simulink model "modello"  (R2023b)
settings: Solver=VariableStepAuto  StartTime=0.0  StopTime=150  RelTol=1e-3
undefined symbols (not defined in the file or in its folder): properties
libraries: fl_lib x60, nesl_utility x27, simulink x1
settings Model: Creator=brent  LastModifiedBy=brent

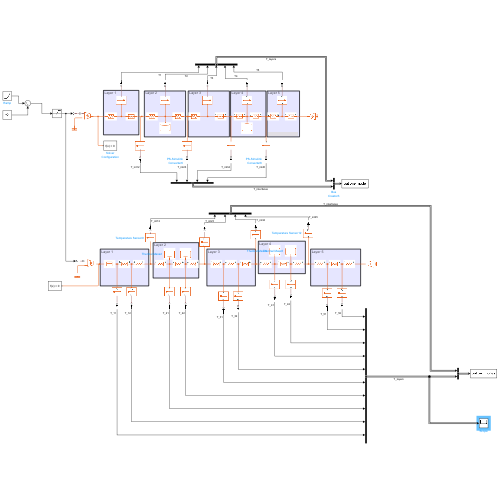
[thumbnail: Simulink's stored preview of the top-level diagram]
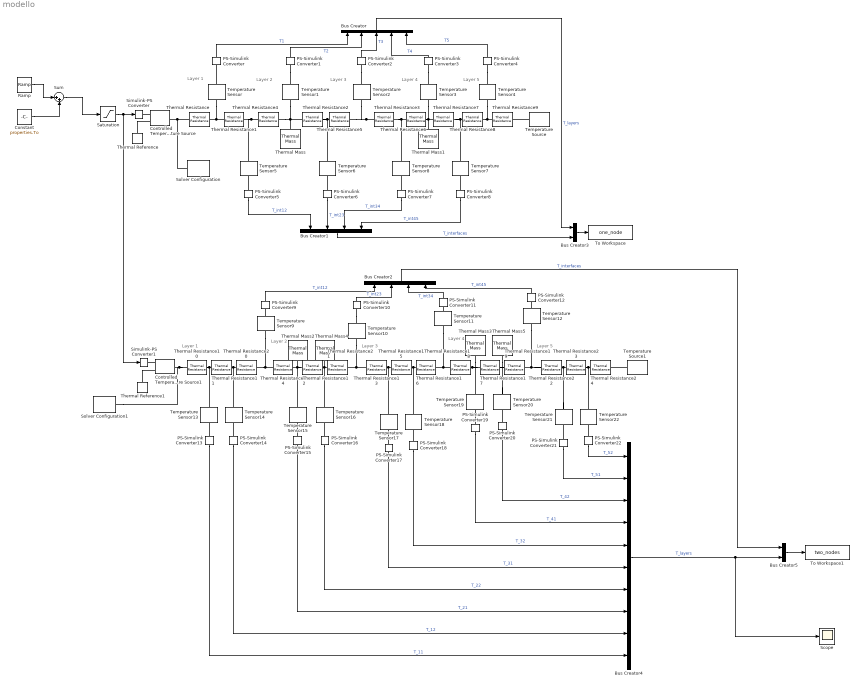
== system modello ==
  note: Layer 1
  note: Layer 2
  note: Layer 1
  note: Layer 3
  note: Layer 4
  note: Layer 5
  note: Layer 2
  note: Layer 3
  note: Layer 4
  note: Layer 5
  Bus Creator : BusCreator  Inputs=5
  Bus Creator1 : BusCreator  Inputs=4
  Bus Creator2 : BusCreator  Inputs=4
  Bus Creator3 : BusCreator  Inputs=2
  Bus Creator4 : BusCreator  Inputs=10
  Bus Creator5 : BusCreator  Inputs=2
  Constant : Constant  Value=properties.To
  Controlled Temperature Source : fl_lib/Thermal/Thermal Sources/Controlled Temperature Source
  Controlled Temperature Source1 : fl_lib/Thermal/Thermal Sources/Controlled Temperature Source
  PS-Simulink Converter{,1..22} (23 alike) : nesl_utility/PS-Simulink Converter  PhysicalDomain=network_engine_domain  SubClassName=ps_output  LeftPortType=input  RightPortType=output  PseudoPeriodic=off  Frequencies=[]  VectorFormat=inherit  Unit=inherit  AffineConversion=off
  Ramp : simulink/Sources/Ramp  slope=980+ 273.15  start=0  InitialOutput=0
  Saturation : Saturate  UpperLimit=1273.15  LowerLimit=273
  Scope : Scope
  Simulink-PS Converter : nesl_utility/Simulink-PS Converter  PhysicalDomain=network_engine_domain  SubClassName=ps_input  LeftPortType=input  RightPortType=output  PseudoPeriodic=off  Frequencies=[]  NoiseDistribution=none  NoiseParameters=[]  Unit=1  AffineConversion=off  FilteringAndDerivatives=provide  SimscapeFilterOrder=1  InputFilterTimeConstant=0.001  UdotUserProvided=0
  Simulink-PS Converter1 : nesl_utility/Simulink-PS Converter  PhysicalDomain=network_engine_domain  SubClassName=ps_input  LeftPortType=input  RightPortType=output  PseudoPeriodic=off  Frequencies=[]  NoiseDistribution=none  NoiseParameters=[]  Unit=1  AffineConversion=off  FilteringAndDerivatives=provide  SimscapeFilterOrder=1  InputFilterTimeConstant=0.001  UdotUserProvided=0
  Solver Configuration : nesl_utility/Solver Configuration  PhysicalDomain=network_engine_domain  SubClassName=solver  LeftPortType=input  RightPortType=generic  Tones=[]  Harmonics=[]  SimulateNoise=off  Profile=off  UseLocalSampling=off  EnableSwitchedLinearOptims=on  FrequencyDomain=off  UseCCode=off  RelTol=0.001  AbsTol=0.001  MinStep=1e-09  ToWorkspace=off  RevertToSquareIcSolve=off  NumHomotopyIterations=100  PhasorMode=off  PhasorModeNumHarmonics=1  ConsistencySolver=NEWTON_XTOL_AFTER_FTOL  IndexReductionMethod=DerivativeReplacement  DoDC=on  ResidualTolerance=1e-09  ConsistencyTolSource=GLOBAL  ConsistencyAbsTol=0.001  ConsistencyRelTol=0.001  ConsistencyTolFactor=ode_tol  UseLocalSolver=off  LocalSolverChoice=NE_BACKWARD_EULER_ADVANCER  ResolveIndetEquations=on  FunctionEvalNumThread=1  LocalSolverSampleTime=0.001  DoFixedCost=off  MaxNonlinIter=3  MaxModeIter=2  ComputeImpulses=off  ImpulseIterations=2  LinearAlgebra=auto  LinearAlgebraNumThread=0  EquationFormulation=NE_TIME_EF  DelaysMemoryBudget=1024  AutomaticFiltering=off  FilteringTimeConstant=0.001  PartitionStorageMethod=AS_NEEDED  PartitionMemoryBudget=1024  PartitionMethod=ROBUST  MultibodyUseLocalSolver=off  MultibodyLocalSolverChoice=ODE1  MultibodyLocalSolverSampleTime=0.001
  Solver Configuration1 : nesl_utility/Solver Configuration  PhysicalDomain=network_engine_domain  SubClassName=solver  LeftPortType=input  RightPortType=generic  Tones=[]  Harmonics=[]  SimulateNoise=off  Profile=off  UseLocalSampling=off  EnableSwitchedLinearOptims=on  FrequencyDomain=off  UseCCode=off  RelTol=0.001  AbsTol=0.001  MinStep=1e-09  ToWorkspace=off  RevertToSquareIcSolve=off  NumHomotopyIterations=100  PhasorMode=off  PhasorModeNumHarmonics=1  ConsistencySolver=NEWTON_XTOL_AFTER_FTOL  IndexReductionMethod=DerivativeReplacement  DoDC=on  ResidualTolerance=1e-09  ConsistencyTolSource=GLOBAL  ConsistencyAbsTol=0.001  ConsistencyRelTol=0.001  ConsistencyTolFactor=ode_tol  UseLocalSolver=off  LocalSolverChoice=NE_BACKWARD_EULER_ADVANCER  ResolveIndetEquations=on  FunctionEvalNumThread=1  LocalSolverSampleTime=0.001  DoFixedCost=off  MaxNonlinIter=3  MaxModeIter=2  ComputeImpulses=off  ImpulseIterations=2  LinearAlgebra=auto  LinearAlgebraNumThread=0  EquationFormulation=NE_TIME_EF  DelaysMemoryBudget=1024  AutomaticFiltering=off  FilteringTimeConstant=0.001  PartitionStorageMethod=AS_NEEDED  PartitionMemoryBudget=1024  PartitionMethod=ROBUST  MultibodyUseLocalSolver=off  MultibodyLocalSolverChoice=ODE1  MultibodyLocalSolverSampleTime=0.001
  Sum : Sum  Inputs=|++
  Temperature Sensor{,1..22} (23 alike) : fl_lib/Thermal/Thermal Sensors/Temperature Sensor  temperature_measure=foundation.enum.MeasurementReference.absolute
      settings: InternalSimscapePortConfiguration="{\"Bottom\":[],\"Left\":[{\"id\":\"A\",\"label\":\"A\",\"type\":\"foundation.thermal.thermal\"}],\"Right\":[{\"id\":\"T\",\"label\":\"T\",\"type\":\"output\"}],\"Top\":[]}"
  Temperature Source : fl_lib/Thermal/Thermal Sources/Temperature Source  temperature=293.15 K
  Temperature Source1 : fl_lib/Thermal/Thermal Sources/Temperature Source  temperature=293.15 K
  Thermal Mass : fl_lib/Thermal/Thermal Elements/Thermal Mass  mass_type=foundation.enum.constant_variable.constant  mass=1 kg  sp_heat=properties.C2 J/(K*kg)  mass_min=1e-6 kg  num_ports=foundation.enum.numPorts2.one  m_specify=off  m_priority=High  m=1 kg  m_nominal_specify=off  m_nominal_unit=kg  m_nominal_value=1  T_specify=off  T_priority=High  T=300 K  T_nominal_specify=off  T_nominal_unit=K  T_nominal_value=1  Q_specify=off  Q_priority=None  Q=0 W  Q_nominal_specify=off  Q_nominal_unit=W  Q_nominal_value=1
  Thermal Mass1 : fl_lib/Thermal/Thermal Elements/Thermal Mass  mass_type=foundation.enum.constant_variable.constant  mass=1 kg  sp_heat=properties.C4 J/(K*kg)  mass_min=1e-6 kg  num_ports=foundation.enum.numPorts2.one  m_specify=off  m_priority=High  m=1 kg  m_nominal_specify=off  m_nominal_unit=kg  m_nominal_value=1  T_specify=off  T_priority=High  T=300 K  T_nominal_specify=off  T_nominal_unit=K  T_nominal_value=1  Q_specify=off  Q_priority=None  Q=0 W  Q_nominal_specify=off  Q_nominal_unit=W  Q_nominal_value=1
  Thermal Mass2 : fl_lib/Thermal/Thermal Elements/Thermal Mass  mass_type=foundation.enum.constant_variable.constant  mass=1 kg  sp_heat=properties.C2/2 J/(K*kg)  mass_min=1e-6 kg  num_ports=foundation.enum.numPorts2.one  m_specify=off  m_priority=High  m=1 kg  m_nominal_specify=off  m_nominal_unit=kg  m_nominal_value=1  T_specify=off  T_priority=High  T=300 K  T_nominal_specify=off  T_nominal_unit=K  T_nominal_value=1  Q_specify=off  Q_priority=None  Q=0 W  Q_nominal_specify=off  Q_nominal_unit=W  Q_nominal_value=1
  Thermal Mass3 : fl_lib/Thermal/Thermal Elements/Thermal Mass  mass_type=foundation.enum.constant_variable.constant  mass=1 kg  sp_heat=properties.C4/2 J/(K*kg)  mass_min=1e-6 kg  num_ports=foundation.enum.numPorts2.one  m_specify=off  m_priority=High  m=1 kg  m_nominal_specify=off  m_nominal_unit=kg  m_nominal_value=1  T_specify=off  T_priority=High  T=300 K  T_nominal_specify=off  T_nominal_unit=K  T_nominal_value=1  Q_specify=off  Q_priority=None  Q=0 W  Q_nominal_specify=off  Q_nominal_unit=W  Q_nominal_value=1
  Thermal Mass4 : fl_lib/Thermal/Thermal Elements/Thermal Mass  mass_type=foundation.enum.constant_variable.constant  mass=1 kg  sp_heat=properties.C2/2 J/(K*kg)  mass_min=1e-6 kg  num_ports=foundation.enum.numPorts2.one  m_specify=off  m_priority=High  m=1 kg  m_nominal_specify=off  m_nominal_unit=kg  m_nominal_value=1  T_specify=off  T_priority=High  T=300 K  T_nominal_specify=off  T_nominal_unit=K  T_nominal_value=1  Q_specify=off  Q_priority=None  Q=0 W  Q_nominal_specify=off  Q_nominal_unit=W  Q_nominal_value=1
  Thermal Mass5 : fl_lib/Thermal/Thermal Elements/Thermal Mass  mass_type=foundation.enum.constant_variable.constant  mass=1 kg  sp_heat=properties.C4/2 J/(K*kg)  mass_min=1e-6 kg  num_ports=foundation.enum.numPorts2.one  m_specify=off  m_priority=High  m=1 kg  m_nominal_specify=off  m_nominal_unit=kg  m_nominal_value=1  T_specify=off  T_priority=High  T=300 K  T_nominal_specify=off  T_nominal_unit=K  T_nominal_value=1  Q_specify=off  Q_priority=None  Q=0 W  Q_nominal_specify=off  Q_nominal_unit=W  Q_nominal_value=1
  Thermal Reference : fl_lib/Thermal/Thermal Elements/Thermal Reference
  Thermal Reference1 : fl_lib/Thermal/Thermal Elements/Thermal Reference
  Thermal Resistance : fl_lib/Thermal/Thermal Elements/Thermal Resistance  resistance=properties.R1/2 K/W  T_specify=off  T_priority=None  T=0 K  T_nominal_specify=off  T_nominal_unit=K  T_nominal_value=1  Q_specify=off  Q_priority=None  Q=0 W  Q_nominal_specify=off  Q_nominal_unit=W  Q_nominal_value=1
  Thermal Resistance1 : fl_lib/Thermal/Thermal Elements/Thermal Resistance  resistance=properties.R1/2 K/W  T_specify=off  T_priority=None  T=0 K  T_nominal_specify=off  T_nominal_unit=K  T_nominal_value=1  Q_specify=off  Q_priority=None  Q=0 W  Q_nominal_specify=off  Q_nominal_unit=W  Q_nominal_value=1
  Thermal Resistance10 : fl_lib/Thermal/Thermal Elements/Thermal Resistance  resistance=properties.R1/3 K/W  T_specify=off  T_priority=None  T=0 K  T_nominal_specify=off  T_nominal_unit=K  T_nominal_value=1  Q_specify=off  Q_priority=None  Q=0 W  Q_nominal_specify=off  Q_nominal_unit=W  Q_nominal_value=1
  Thermal Resistance11 : fl_lib/Thermal/Thermal Elements/Thermal Resistance  resistance=properties.R1/3 K/W  T_specify=off  T_priority=None  T=0 K  T_nominal_specify=off  T_nominal_unit=K  T_nominal_value=1  Q_specify=off  Q_priority=None  Q=0 W  Q_nominal_specify=off  Q_nominal_unit=W  Q_nominal_value=1
  Thermal Resistance12 : fl_lib/Thermal/Thermal Elements/Thermal Resistance  resistance=properties.R2/3 K/W  T_specify=off  T_priority=None  T=0 K  T_nominal_specify=off  T_nominal_unit=K  T_nominal_value=1  Q_specify=off  Q_priority=None  Q=0 W  Q_nominal_specify=off  Q_nominal_unit=W  Q_nominal_value=1
  Thermal Resistance13 : fl_lib/Thermal/Thermal Elements/Thermal Resistance  resistance=properties.R3/3 K/W  T_specify=off  T_priority=None  T=0 K  T_nominal_specify=off  T_nominal_unit=K  T_nominal_value=1  Q_specify=off  Q_priority=None  Q=0 W  Q_nominal_specify=off  Q_nominal_unit=W  Q_nominal_value=1
  Thermal Resistance14 : fl_lib/Thermal/Thermal Elements/Thermal Resistance  resistance=properties.R2/3 K/W  T_specify=off  T_priority=None  T=0 K  T_nominal_specify=off  T_nominal_unit=K  T_nominal_value=1  Q_specify=off  Q_priority=None  Q=0 W  Q_nominal_specify=off  Q_nominal_unit=W  Q_nominal_value=1
  Thermal Resistance15 : fl_lib/Thermal/Thermal Elements/Thermal Resistance  resistance=properties.R3/3 K/W  T_specify=off  T_priority=None  T=0 K  T_nominal_specify=off  T_nominal_unit=K  T_nominal_value=1  Q_specify=off  Q_priority=None  Q=0 W  Q_nominal_specify=off  Q_nominal_unit=W  Q_nominal_value=1
  Thermal Resistance16 : fl_lib/Thermal/Thermal Elements/Thermal Resistance  resistance=properties.R3/3 K/W  T_specify=off  T_priority=None  T=0 K  T_nominal_specify=off  T_nominal_unit=K  T_nominal_value=1  Q_specify=off  Q_priority=None  Q=0 W  Q_nominal_specify=off  Q_nominal_unit=W  Q_nominal_value=1
  Thermal Resistance17 : fl_lib/Thermal/Thermal Elements/Thermal Resistance  resistance=properties.R4/3 K/W  T_specify=off  T_priority=None  T=0 K  T_nominal_specify=off  T_nominal_unit=K  T_nominal_value=1  Q_specify=off  Q_priority=None  Q=0 W  Q_nominal_specify=off  Q_nominal_unit=W  Q_nominal_value=1
  Thermal Resistance18 : fl_lib/Thermal/Thermal Elements/Thermal Resistance  resistance=properties.R4/3 K/W  T_specify=off  T_priority=None  T=0 K  T_nominal_specify=off  T_nominal_unit=K  T_nominal_value=1  Q_specify=off  Q_priority=None  Q=0 W  Q_nominal_specify=off  Q_nominal_unit=W  Q_nominal_value=1
  Thermal Resistance19 : fl_lib/Thermal/Thermal Elements/Thermal Resistance  resistance=properties.R4/3 K/W  T_specify=off  T_priority=None  T=0 K  T_nominal_specify=off  T_nominal_unit=K  T_nominal_value=1  Q_specify=off  Q_priority=None  Q=0 W  Q_nominal_specify=off  Q_nominal_unit=W  Q_nominal_value=1
  Thermal Resistance2 : fl_lib/Thermal/Thermal Elements/Thermal Resistance  resistance=properties.R2/2 K/W  T_specify=off  T_priority=None  T=0 K  T_nominal_specify=off  T_nominal_unit=K  T_nominal_value=1  Q_specify=off  Q_priority=None  Q=0 W  Q_nominal_specify=off  Q_nominal_unit=W  Q_nominal_value=1
  Thermal Resistance20 : fl_lib/Thermal/Thermal Elements/Thermal Resistance  resistance=properties.R1/3 K/W  T_specify=off  T_priority=None  T=0 K  T_nominal_specify=off  T_nominal_unit=K  T_nominal_value=1  Q_specify=off  Q_priority=None  Q=0 W  Q_nominal_specify=off  Q_nominal_unit=W  Q_nominal_value=1
  Thermal Resistance21 : fl_lib/Thermal/Thermal Elements/Thermal Resistance  resistance=properties.R2/3 K/W  T_specify=off  T_priority=None  T=0 K  T_nominal_specify=off  T_nominal_unit=K  T_nominal_value=1  Q_specify=off  Q_priority=None  Q=0 W  Q_nominal_specify=off  Q_nominal_unit=W  Q_nominal_value=1
  Thermal Resistance22 : fl_lib/Thermal/Thermal Elements/Thermal Resistance  resistance=properties.R5/3 K/W  T_specify=off  T_priority=None  T=0 K  T_nominal_specify=off  T_nominal_unit=K  T_nominal_value=1  Q_specify=off  Q_priority=None  Q=0 W  Q_nominal_specify=off  Q_nominal_unit=W  Q_nominal_value=1
  Thermal Resistance23 : fl_lib/Thermal/Thermal Elements/Thermal Resistance  resistance=properties.R5/3 K/W  T_specify=off  T_priority=None  T=0 K  T_nominal_specify=off  T_nominal_unit=K  T_nominal_value=1  Q_specify=off  Q_priority=None  Q=0 W  Q_nominal_specify=off  Q_nominal_unit=W  Q_nominal_value=1
  Thermal Resistance24 : fl_lib/Thermal/Thermal Elements/Thermal Resistance  resistance=properties.R5/3 K/W  T_specify=off  T_priority=None  T=0 K  T_nominal_specify=off  T_nominal_unit=K  T_nominal_value=1  Q_specify=off  Q_priority=None  Q=0 W  Q_nominal_specify=off  Q_nominal_unit=W  Q_nominal_value=1
  Thermal Resistance3 : fl_lib/Thermal/Thermal Elements/Thermal Resistance  resistance=properties.R3/2 K/W  T_specify=off  T_priority=None  T=0 K  T_nominal_specify=off  T_nominal_unit=K  T_nominal_value=1  Q_specify=off  Q_priority=None  Q=0 W  Q_nominal_specify=off  Q_nominal_unit=W  Q_nominal_value=1
  Thermal Resistance4 : fl_lib/Thermal/Thermal Elements/Thermal Resistance  resistance=properties.R2/2 K/W  T_specify=off  T_priority=None  T=0 K  T_nominal_specify=off  T_nominal_unit=K  T_nominal_value=1  Q_specify=off  Q_priority=None  Q=0 W  Q_nominal_specify=off  Q_nominal_unit=W  Q_nominal_value=1
  Thermal Resistance5 : fl_lib/Thermal/Thermal Elements/Thermal Resistance  resistance=properties.R3/2 K/W  T_specify=off  T_priority=None  T=0 K  T_nominal_specify=off  T_nominal_unit=K  T_nominal_value=1  Q_specify=off  Q_priority=None  Q=0 W  Q_nominal_specify=off  Q_nominal_unit=W  Q_nominal_value=1
  Thermal Resistance6 : fl_lib/Thermal/Thermal Elements/Thermal Resistance  resistance=properties.R4/2 K/W  T_specify=off  T_priority=None  T=0 K  T_nominal_specify=off  T_nominal_unit=K  T_nominal_value=1  Q_specify=off  Q_priority=None  Q=0 W  Q_nominal_specify=off  Q_nominal_unit=W  Q_nominal_value=1
  Thermal Resistance7 : fl_lib/Thermal/Thermal Elements/Thermal Resistance  resistance=properties.R4/2 K/W  T_specify=off  T_priority=None  T=0 K  T_nominal_specify=off  T_nominal_unit=K  T_nominal_value=1  Q_specify=off  Q_priority=None  Q=0 W  Q_nominal_specify=off  Q_nominal_unit=W  Q_nominal_value=1
  Thermal Resistance8 : fl_lib/Thermal/Thermal Elements/Thermal Resistance  resistance=properties.R5/2 K/W  T_specify=off  T_priority=None  T=0 K  T_nominal_specify=off  T_nominal_unit=K  T_nominal_value=1  Q_specify=off  Q_priority=None  Q=0 W  Q_nominal_specify=off  Q_nominal_unit=W  Q_nominal_value=1
  Thermal Resistance9 : fl_lib/Thermal/Thermal Elements/Thermal Resistance  resistance=properties.R5/2 K/W  T_specify=off  T_priority=None  T=0 K  T_nominal_specify=off  T_nominal_unit=K  T_nominal_value=1  Q_specify=off  Q_priority=None  Q=0 W  Q_nominal_specify=off  Q_nominal_unit=W  Q_nominal_value=1
  To Workspace : ToWorkspace  VariableName=one_node  SaveFormat=Timeseries  SampleTime=-1
  To Workspace1 : ToWorkspace  VariableName=two_nodes  SaveFormat=Timeseries  SampleTime=-1
  wires:
  Ramp/1 -> Sum/1
  Constant/1 -> Sum/2
  Sum/1 -> Saturation/1
  Saturation/1 -> Simulink-PS Converter1/1, Simulink-PS Converter/1
  Bus Creator/1 -> Bus Creator3/1  "T_layers"
  PS-Simulink Converter/1 -> Bus Creator/1  "T1"
  PS-Simulink Converter1/1 -> Bus Creator/2  "T2"
  PS-Simulink Converter2/1 -> Bus Creator/3  "T3"
  PS-Simulink Converter3/1 -> Bus Creator/4  "T4"
  PS-Simulink Converter4/1 -> Bus Creator/5  "T5"
  PS-Simulink Converter5/1 -> Bus Creator1/1  "T_int12"
  PS-Simulink Converter6/1 -> Bus Creator1/2  "T_int23"
  PS-Simulink Converter8/1 -> Bus Creator1/4  "T_int45"
  PS-Simulink Converter7/1 -> Bus Creator1/3  "T_int34"
  PS-Simulink Converter10/1 -> Bus Creator2/2  "T_int23"
  PS-Simulink Converter9/1 -> Bus Creator2/1  "T_int12"
  PS-Simulink Converter11/1 -> Bus Creator2/3  "T_int34"
  PS-Simulink Converter12/1 -> Bus Creator2/4  "T_int45"
  Bus Creator1/1 -> Bus Creator3/2  "T_interfaces"
  Bus Creator2/1 -> Bus Creator5/1  "T_interfaces"
  Bus Creator3/1 -> To Workspace/1
  PS-Simulink Converter22/1 -> Bus Creator4/1  "T_52"
  PS-Simulink Converter21/1 -> Bus Creator4/2  "T_51"
  PS-Simulink Converter20/1 -> Bus Creator4/3  "T_42"
  PS-Simulink Converter19/1 -> Bus Creator4/4  "T_41"
  PS-Simulink Converter18/1 -> Bus Creator4/5  "T_32"
  PS-Simulink Converter17/1 -> Bus Creator4/6  "T_31"
  PS-Simulink Converter16/1 -> Bus Creator4/7  "T_22"
  PS-Simulink Converter15/1 -> Bus Creator4/8  "T_21"
  PS-Simulink Converter14/1 -> Bus Creator4/9  "T_12"
  PS-Simulink Converter13/1 -> Bus Creator4/10  "T_11"
  Bus Creator4/1 -> Scope/1, Bus Creator5/2  "T_layers"
  Bus Creator5/1 -> To Workspace1/1
  connections:
  Thermal Resistance1/LConn1 -- Temperature Sensor/LConn1 -- Thermal Resistance/RConn1
  Thermal Resistance4/LConn1 -- Temperature Sensor5/LConn1 -- Thermal Resistance1/RConn1
  Thermal Resistance4/RConn1 -- Temperature Sensor1/LConn1 -- Thermal Mass/LConn1 -- Thermal Resistance2/LConn1
  Thermal Resistance3/LConn1 -- Temperature Sensor2/LConn1 -- Thermal Resistance5/RConn1
  Thermal Resistance5/LConn1 -- Temperature Sensor6/LConn1 -- Thermal Resistance2/RConn1
  Thermal Resistance7/LConn1 -- Thermal Mass1/LConn1 -- Temperature Sensor3/LConn1 -- Thermal Resistance6/RConn1
  Thermal Resistance6/LConn1 -- Temperature Sensor8/LConn1 -- Thermal Resistance3/RConn1
  Thermal Resistance9/LConn1 -- Temperature Sensor4/LConn1 -- Thermal Resistance8/RConn1
  Thermal Resistance8/LConn1 -- Temperature Sensor7/LConn1 -- Thermal Resistance7/RConn1
  Temperature Source/LConn1 -- Thermal Resistance9/RConn1
  Controlled Temperature Source/LConn1 -- Thermal Resistance/LConn1 -- Solver Configuration/RConn1
  Simulink-PS Converter/RConn1 -- Controlled Temperature Source/RConn1
  Temperature Sensor/RConn1 -- PS-Simulink Converter/LConn1
  PS-Simulink Converter1/LConn1 -- Temperature Sensor1/RConn1
  Thermal Reference/LConn1 -- Controlled Temperature Source/RConn2
  PS-Simulink Converter2/LConn1 -- Temperature Sensor2/RConn1
  PS-Simulink Converter3/LConn1 -- Temperature Sensor3/RConn1
  PS-Simulink Converter4/LConn1 -- Temperature Sensor4/RConn1
  Thermal Resistance14/RConn1 -- Temperature Sensor15/LConn1 -- Thermal Mass2/LConn1 -- Thermal Resistance12/LConn1
  Thermal Resistance11/LConn1 -- Temperature Sensor13/LConn1 -- Thermal Resistance10/RConn1
  Controlled Temperature Source1/LConn1 -- Solver Configuration1/RConn1 -- Thermal Resistance10/LConn1
  Thermal Reference1/LConn1 -- Controlled Temperature Source1/RConn2
  Simulink-PS Converter1/RConn1 -- Controlled Temperature Source1/RConn1
  Thermal Resistance20/LConn1 -- Temperature Sensor14/LConn1 -- Thermal Resistance11/RConn1
  Thermal Resistance20/RConn1 -- Temperature Sensor9/LConn1 -- Thermal Resistance14/LConn1
  Thermal Resistance21/LConn1 -- Temperature Sensor16/LConn1 -- Thermal Mass4/LConn1 -- Thermal Resistance12/RConn1
  Thermal Resistance13/LConn1 -- Temperature Sensor10/LConn1 -- Thermal Resistance21/RConn1
  Thermal Resistance15/LConn1 -- Temperature Sensor17/LConn1 -- Thermal Resistance13/RConn1
  Thermal Resistance16/LConn1 -- Temperature Sensor18/LConn1 -- Thermal Resistance15/RConn1
  Thermal Resistance17/LConn1 -- Temperature Sensor19/LConn1 -- Thermal Mass3/LConn1 -- Thermal Resistance18/RConn1
  Thermal Resistance17/RConn1 -- Temperature Sensor20/LConn1 -- Thermal Mass5/LConn1 -- Thermal Resistance19/LConn1
  Thermal Resistance16/RConn1 -- Temperature Sensor11/LConn1 -- Thermal Resistance18/LConn1
  Thermal Resistance22/LConn1 -- Temperature Sensor12/LConn1 -- Thermal Resistance19/RConn1
  Temperature Source1/LConn1 -- Thermal Resistance24/RConn1
  Thermal Resistance24/LConn1 -- Temperature Sensor22/LConn1 -- Thermal Resistance23/RConn1
  Thermal Resistance23/LConn1 -- Temperature Sensor21/LConn1 -- Thermal Resistance22/RConn1
  PS-Simulink Converter8/LConn1 -- Temperature Sensor7/RConn1
  PS-Simulink Converter7/LConn1 -- Temperature Sensor8/RConn1
  PS-Simulink Converter6/LConn1 -- Temperature Sensor6/RConn1
  PS-Simulink Converter5/LConn1 -- Temperature Sensor5/RConn1
  PS-Simulink Converter9/LConn1 -- Temperature Sensor9/RConn1
  PS-Simulink Converter10/LConn1 -- Temperature Sensor10/RConn1
  PS-Simulink Converter11/LConn1 -- Temperature Sensor11/RConn1
  PS-Simulink Converter12/LConn1 -- Temperature Sensor12/RConn1
  PS-Simulink Converter13/LConn1 -- Temperature Sensor13/RConn1
  PS-Simulink Converter14/LConn1 -- Temperature Sensor14/RConn1
  PS-Simulink Converter15/LConn1 -- Temperature Sensor15/RConn1
  PS-Simulink Converter16/LConn1 -- Temperature Sensor16/RConn1
  PS-Simulink Converter18/LConn1 -- Temperature Sensor18/RConn1
  PS-Simulink Converter17/LConn1 -- Temperature Sensor17/RConn1
  PS-Simulink Converter20/LConn1 -- Temperature Sensor20/RConn1
  PS-Simulink Converter19/LConn1 -- Temperature Sensor19/RConn1
  PS-Simulink Converter22/LConn1 -- Temperature Sensor22/RConn1
  PS-Simulink Converter21/LConn1 -- Temperature Sensor21/RConn1
